simulink model "Lab6SNL"  (R2018a)
settings: Solver=VariableStepAuto  StartTime=0.0  StopTime=50.0  MaxStep=0.001  RelTol=1e-3
values from neighbouring files (symbols this model uses):
  A1 = k(1)    [Lab6-2.m]
  A2 = k(1)    [Lab6-2.m]
  Aw1 = 0.1 * k(1)    [Lab6-2.m]
  Aw2 = 0.1 * k(1)    [Lab6-2.m]
  delay = 10    [Lab6-2.m]
  Fw1 = FWe10(i)    [Lab6-2.m]
  FW1max = Aw1 * sqrt( 2 * g * ( H1max - H2max ) )    [Lab6-2.m]
  Fw2 = FWe20(i)    [Lab6-2.m]
  FW2max = Aw2 * sqrt( 2 * g * H2max ) - 0    [Lab6-2.m]
  g = 9.81    [Lab6-2.m]
  H10NL = Fw1^2/(2*Aw1^2*g) + H20NL    [Lab6-2.m]
  H20NL = ((Fw1 + Fw2)^2) / (2*(Aw2^2)*g)    [Lab6-2.m]
settings Model: Creator=aplov  LastModifiedBy=aplov

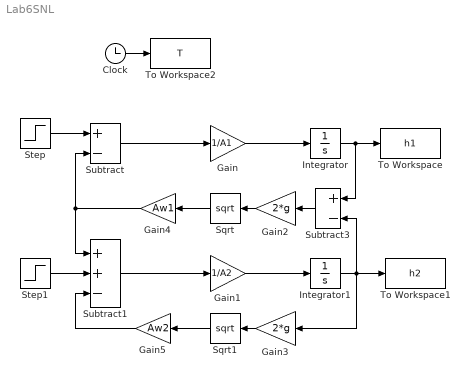
== system Lab6SNL ==
  Clock : Clock
  Gain : Gain  Gain=1/A1
  Gain1 : Gain  Gain=1/A2
  Gain2 : Gain  Gain=2*g
  Gain3 : Gain  Gain=2*g
  Gain4 : Gain  Gain=Aw1
  Gain5 : Gain  Gain=Aw2
  Integrator : Integrator  InitialCondition=H10NL
  Integrator1 : Integrator  InitialCondition=H20NL
  Sqrt : Sqrt  SaturateOnIntegerOverflow=on
  Sqrt1 : Sqrt  SaturateOnIntegerOverflow=on
  Step : Step  Time=delay  Before=Fw1  After=Fw1 + 0.1*FW1max  SampleTime=0
  Step1 : Step  Time=delay  Before=Fw2  After=Fw2 + FW2max  SampleTime=0
  Subtract : Sum  Inputs=+-
  Subtract1 : Sum  Inputs=++-
  Subtract3 : Sum  Inputs=+-
  To Workspace : ToWorkspace  VariableName=h1  SampleTime=-1
  To Workspace1 : ToWorkspace  VariableName=h2  SampleTime=-1
  To Workspace2 : ToWorkspace  VariableName=T  SampleTime=-1
  wires:
  Step/1 -> Subtract/1
  Subtract/1 -> Gain/1
  Gain/1 -> Integrator/1
  Integrator/1 -> Subtract3/1, To Workspace/1
  Subtract1/1 -> Gain1/1
  Gain1/1 -> Integrator1/1
  Subtract3/1 -> Gain2/1
  Integrator1/1 -> Gain3/1, Subtract3/2, To Workspace1/1
  Step1/1 -> Subtract1/2
  Clock/1 -> To Workspace2/1
  Sqrt1/1 -> Gain5/1
  Sqrt/1 -> Gain4/1
  Gain3/1 -> Sqrt1/1
  Gain2/1 -> Sqrt/1
  Gain4/1 -> Subtract/2, Subtract1/1
  Gain5/1 -> Subtract1/3
